simulink model "SlidingModeRobot"  (R2015b)
settings: Solver=ode4  StartTime=0.0  StopTime=20  FixedStep=0.01  RelTol=1e-3
InitFcn:
  | Set_Parameter
StopFcn:
  | Draw_7DOF_FB7roll_point_script
  | DrawResult
values from neighbouring files (symbols this model uses):
  b = 0.1    [Set_Parameter.m]    (also in Set_Parameter_Single.m; Set_Parameter_line_circle.m; Set_Parameter_line_circle_DC_model_no_vision_controller.m; Set_Parameter_sewing_DC_model_no_vision_controller.m)
  J = 0.01    [Set_Parameter.m]    (also in Set_Parameter_Single.m = [0.016,0.016,0.012,0.012,0.01,0.01,0.01]; Set_Parameter_line_circle.m = [0.016,0.016,0.012,0.012,0.01,0.01,0.01]; Set_Parameter_line_circle_DC_model_no_vision_controller.m = [0.016,0.016,0.012,0.012,0.01,0.01,0.01]; Set_Parameter_line_circle_no_vision_controller.m = [10,10,8,8,4,4,4])
  K = 0.01    [Set_Parameter.m]    (also in Set_Parameter_Single.m; Set_Parameter_line_circle.m; Set_Parameter_line_circle_DC_model_no_vision_controller.m; Set_Parameter_sewing_DC_model_no_vision_controller.m)
  L = 0.5    [Set_Parameter.m]    (also in Set_Parameter_Single.m; Set_Parameter_line_circle.m; Set_Parameter_line_circle_DC_model_no_vision_controller.m; Set_Parameter_sewing_DC_model_no_vision_controller.m)
  R = R_z1x2y3(PoseAngle(1),PoseAngle(2),PoseAngle(3))    [IK_7DOF_FB7roll.m]    (also in Set_Parameter.m = 1; Set_Parameter_Single.m = 1; Set_Parameter_line_circle.m = 1; Set_Parameter_line_circle_DC_model_no_vision_controller.m = 1)
undefined symbols (not defined in the file or in its folder): IniJointAngle
libraries: simulink x14
settings Model: Creator=User  LastModifiedBy=User

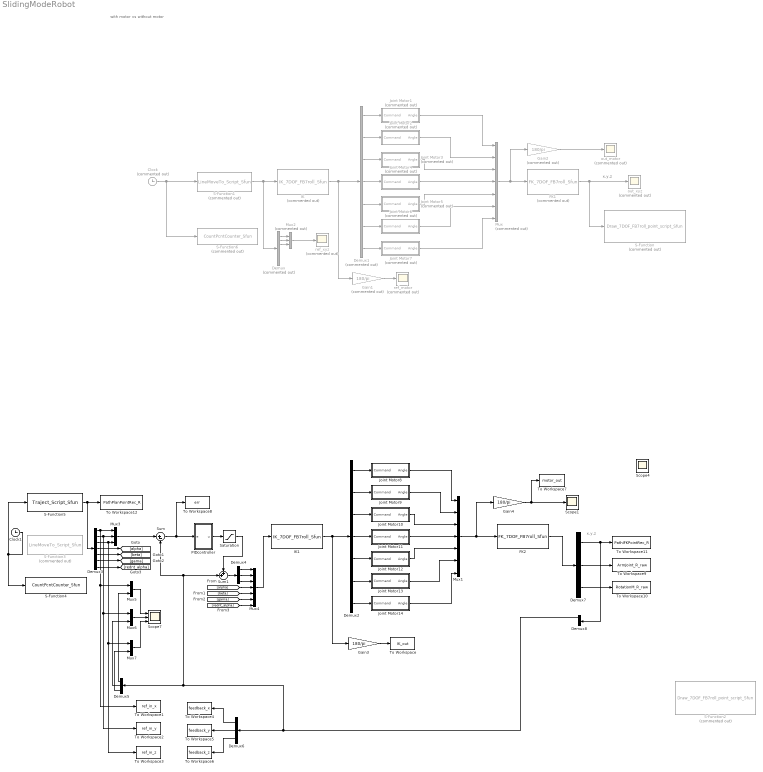
== system SlidingModeRobot ==
  note: with motor vs without motor
  note: x,y,z
  note: x,y,z
  Clock : Clock  Commented=on
  Clock1 : Clock
  Demux : Demux  Commented=on  Outputs=7
  Demux1 : Demux  Commented=on  Outputs=7
  Demux2 : Demux  Outputs=7
  Demux3 : Demux  Outputs=7
  Demux4 : Demux  Outputs=3
  Demux5 : Demux  Outputs=3
  Demux6 : Demux  Outputs=3
  Demux7 : Demux  Outputs=[7,30,9]
  Demux8 : Demux  Outputs=[3,4]
  FK1 : S-Function  Commented=on  FunctionName=FK_7DOF_FB7roll_Sfun  SFunctionDeploymentMode=off  EnableBusSupport=off
  FK2 : S-Function  FunctionName=FK_7DOF_FB7roll_Sfun  SFunctionDeploymentMode=off  EnableBusSupport=off
  Gain1 : Gain  Commented=on  Gain=180/pi
  Gain2 : Gain  Commented=on  Gain=180/pi
  Gain3 : Gain  Gain=180/pi
  Gain4 : Gain  Gain=180/pi
  IK : S-Function  Commented=on  FunctionName=IK_7DOF_FB7roll_Sfun  SFunctionDeploymentMode=off  EnableBusSupport=off
  IK1 : S-Function  FunctionName=IK_7DOF_FB7roll_Sfun  SFunctionDeploymentMode=off  EnableBusSupport=off
  Joint Motor1 : Subsystem  Commented=on
  Joint Motor10 : Subsystem
  Joint Motor11 : Subsystem
  Joint Motor12 : Subsystem
  Joint Motor13 : Subsystem
  Joint Motor14 : Subsystem
  Joint Motor2 : Subsystem  Commented=on
  Joint Motor3 : Subsystem  Commented=on
  Joint Motor4 : Subsystem  Commented=on
  Joint Motor5 : Subsystem  Commented=on
  Joint Motor6 : Subsystem  Commented=on
  Joint Motor7 : Subsystem  Commented=on
  Joint Motor8 : Subsystem
  Joint Motor9 : Subsystem
  Mux : Mux  Commented=on  Inputs=7
  Mux1 : Mux  Inputs=7
  Mux2 : Mux  Commented=on  Inputs=3
  Mux3 : Mux  Inputs=3
  Mux4 : Mux  Inputs=7
  Mux5 : Mux  Inputs=2
  Mux6 : Mux  Inputs=2
  Mux7 : Mux  Inputs=2
  PIDcontroller : Subsystem
  S-Function : S-Function  Commented=on  FunctionName=Draw_7DOF_FB7roll_point_script_Sfun  SFunctionDeploymentMode=off  EnableBusSupport=off
  S-Function1 : S-Function  Commented=on  FunctionName=LineMoveTo_Script_Sfun  SFunctionDeploymentMode=off  EnableBusSupport=off
  S-Function2 : S-Function  Commented=on  FunctionName=Draw_7DOF_FB7roll_point_script_Sfun  SFunctionDeploymentMode=off  EnableBusSupport=off
  S-Function3 : S-Function  Commented=on  FunctionName=LineMoveTo_Script_Sfun  SFunctionDeploymentMode=off  EnableBusSupport=off
  S-Function4 : S-Function  FunctionName=CountPcntCounter_Sfun  SFunctionDeploymentMode=off  EnableBusSupport=off
  S-Function5 : S-Function  FunctionName=Traject_Script_Sfun  SFunctionDeploymentMode=off  EnableBusSupport=off
  S-Function6 : S-Function  Commented=on  FunctionName=CountPcntCounter_Sfun  SFunctionDeploymentMode=off  EnableBusSupport=off
  Saturation : Saturate  UpperLimit=50  LowerLimit=-50
  Scope1 : Scope
  Scope4 : Scope
  Scope7 : Scope  NumInputPorts=3
  Sum : Sum  Inputs=|+-
  Sum1 : Sum  Inputs=++|
  To Workspace : ToWorkspace  VariableName=IK_out  SaveFormat=Timeseries  SampleTime=-1
  To Workspace1 : ToWorkspace  VariableName=ref_in_x  SaveFormat=Timeseries  SampleTime=-1
  To Workspace10 : ToWorkspace  VariableName=RotationM_R_raw  SaveFormat=Timeseries  SampleTime=-1
  To Workspace11 : ToWorkspace  VariableName=PathIFKPointRec_R  SaveFormat=Timeseries  SampleTime=-1
  To Workspace12 : ToWorkspace  VariableName=PathPlanPointRec_R  SaveFormat=Timeseries  SampleTime=-1
  To Workspace2 : ToWorkspace  VariableName=ref_in_y  SaveFormat=Timeseries  SampleTime=-1
  To Workspace3 : ToWorkspace  VariableName=ref_in_z  SaveFormat=Timeseries  SampleTime=-1
  To Workspace4 : ToWorkspace  VariableName=feedback_x  SaveFormat=Timeseries  SampleTime=-1
  To Workspace5 : ToWorkspace  VariableName=feedback_y  SaveFormat=Timeseries  SampleTime=-1
  To Workspace6 : ToWorkspace  VariableName=feedback_z  SaveFormat=Timeseries  SampleTime=-1
  To Workspace7 : ToWorkspace  VariableName=motor_out  SaveFormat=Timeseries  SampleTime=-1
  To Workspace8 : ToWorkspace  VariableName=err  SaveFormat=Timeseries  SampleTime=-1
  To Workspace9 : ToWorkspace  VariableName=ArmJoint_R_raw  SaveFormat=Timeseries  SampleTime=-1
  out_motor : Scope  Commented=on
  out_xyz : Scope  Commented=on
  ref_motor : Scope  Commented=on
  ref_xyz : Scope  Commented=on
  wires:
  Joint Motor3/1(Angle) -> Mux/3
  Joint Motor1/1(Angle) -> Mux/1
  Joint Motor2/1(Angle) -> Mux/2
  Joint Motor4/1(Angle) -> Mux/4
  Joint Motor5/1(Angle) -> Mux/5
  Joint Motor6/1(Angle) -> Mux/6
  Joint Motor7/1(Angle) -> Mux/7
  S-Function1/1 -> Demux/1, IK/1
  Gain1/1 -> ref_motor/1
  FK1/1 -> S-Function/1, out_xyz/1
  Gain2/1 -> out_motor/1
  Demux1/7 -> Joint Motor7/1(Command)
  Demux1/6 -> Joint Motor6/1(Command)
  Demux1/5 -> Joint Motor5/1(Command)
  Demux1/4 -> Joint Motor4/1(Command)
  Demux1/1 -> Joint Motor1/1(Command)
  Demux1/2 -> Joint Motor2/1(Command)
  Demux1/3 -> Joint Motor3/1(Command)
  IK/1 -> Demux1/1, Gain1/1
  Clock/1 -> S-Function6/1, S-Function1/1
  Mux/1 -> Gain2/1, FK1/1
  Joint Motor10/1(Angle) -> Mux1/3
  Joint Motor8/1(Angle) -> Mux1/1
  Joint Motor9/1(Angle) -> Mux1/2
  Joint Motor11/1(Angle) -> Mux1/4
  Joint Motor12/1(Angle) -> Mux1/5
  Joint Motor13/1(Angle) -> Mux1/6
  Joint Motor14/1(Angle) -> Mux1/7
  Gain3/1 -> To Workspace/1
  Gain4/1 -> To Workspace7/1, Scope1/1
  Demux2/7 -> Joint Motor14/1(Command)
  Demux2/6 -> Joint Motor13/1(Command)
  Demux2/5 -> Joint Motor12/1(Command)
  Demux2/4 -> Joint Motor11/1(Command)
  Demux2/1 -> Joint Motor8/1(Command)
  Demux2/2 -> Joint Motor9/1(Command)
  Demux2/3 -> Joint Motor10/1(Command)
  IK1/1 -> Demux2/1, Gain3/1
  Clock1/1 -> S-Function5/1, S-Function4/1
  Mux1/1 -> Gain4/1, FK2/1
  Sum/1 -> To Workspace8/1, PIDcontroller/1(e)
  Demux/1 -> Mux2/1
  Demux/2 -> Mux2/2
  Demux/3 -> Mux2/3
  Mux2/1 -> ref_xyz/1
  Demux3/1 -> Mux3/1, To Workspace1/1, Mux5/1
  Demux3/2 -> Mux3/2, To Workspace2/1, Mux6/1
  Demux3/3 -> Mux7/1, To Workspace3/1, Mux3/3
  Demux3/4 -> [alpha]
  Demux3/5 -> [beta]
  Demux3/6 -> [gama]
  [gama] -> Mux4/6
  [beta] -> Mux4/5
  [alpha] -> Mux4/4
  Demux4/1 -> Mux4/1
  Demux4/2 -> Mux4/2
  Demux4/3 -> Mux4/3
  Mux4/1 -> IK1/1
  Demux3/7 -> [rednt_alpha]
  [rednt_alpha] -> Mux4/7
  S-Function5/1 -> To Workspace12/1, Demux3/1
  Mux3/1 -> Sum/1
  Demux5/1 -> Mux5/2
  Demux5/2 -> Mux6/2
  Demux5/3 -> Mux7/2
  Mux6/1 -> Scope7/2
  Mux5/1 -> Scope7/1
  Mux7/1 -> Scope7/3
  PIDcontroller/1(u) -> Saturation/1
  Saturation/1 -> Sum1/1
  Sum1/1 -> Demux4/1
  Demux6/1 -> To Workspace4/1
  Demux6/2 -> To Workspace5/1
  Demux6/3 -> To Workspace6/1
  FK2/1 -> Demux7/1
  Demux7/1 -> To Workspace11/1, Demux8/1
  Demux7/2 -> To Workspace9/1
  Demux7/3 -> To Workspace10/1
  Demux8/1 -> Sum1/2, Sum/2, Demux5/1, Demux6/1

== system SlidingModeRobot/Joint Motor1 ==
  Command : Inport
  Constant : Constant  Value=IniJointAngle(1)
  DC motor : Subsystem
  Gain : Gain  Gain=30
  Integrator : Integrator  InitialConditionSource=external
  PID Controller : simulink/Continuous/PID Controller  Controller=PID  TimeDomain=Continuous-time  SampleTime=-1  IntegratorMethod=Forward Euler  FilterMethod=Forward Euler  Form=Parallel  UseFilter=on  ControllerParametersSource=internal  P=20  I=0  D=20  N=0  InitialConditionSource=internal  InitialConditionForIntegrator=0  InitialConditionForFilter=0  ExternalReset=none  LimitOutput=off  UpperSaturationLimit=inf  LowerSaturationLimit=-inf  LinearizeAsGain=on  AntiWindupMode=none  Kb=1  TrackingMode=off  Kt=1  PParamMin=[]  PParamMax=[]  IParamMin=[]  IParamMax=[]  DParamMin=[]  DParamMax=[]  NParamMin=[]  NParamMax=[]  KbParamMin=[]  KbParamMax=[]  KtParamMin=[]  KtParamMax=[]  POutMin=[]  POutMax=[]  IOutMin=[]  IOutMax=[]  DOutMin=[]  DOutMax=[]  NOutMin=[]  NOutMax=[]  KbOutMin=[]  KbOutMax=[]  KtOutMin=[]  KtOutMax=[]  IntegratorOutMin=[]  IntegratorOutMax=[]  FilterOutMin=[]  FilterOutMax=[]  SumOutMin=[]  SumOutMax=[]  SumI1OutMin=[]  SumI1OutMax=[]  SumI2OutMin=[]  SumI2OutMax=[]  SumI3OutMin=[]  SumI3OutMax=[]  SumDOutMin=[]  SumDOutMax=[]  SaturationOutMin=[]  SaturationOutMax=[]  IntegratorContinuousStateAttributes=''  IntegratorStateMustResolveToSignalObject=off  IntegratorRTWStateStorageClass=Auto  FilterContinuousStateAttributes=''  FilterStateMustResolveToSignalObject=off  FilterRTWStateStorageClass=Auto  DifferentiatorICPrevScaledInput=0  DifferentiatorOutMin=[]  DifferentiatorOutMax=[]
  Sum : Sum  Inputs=|+-
  Sum1 : Sum  Inputs=|+-
  Angle : Outport
  wires:
  Sum/1 -> PID Controller/1
  PID Controller/1 -> DC motor/1(Voltage)
  DC motor/1(Speed) -> Sum/2, Integrator/1
  Integrator/1 -> Angle/1, Sum1/2
  Command/1 -> Sum1/1
  Sum1/1 -> Gain/1
  Gain/1 -> Sum/1
  Constant/1 -> Integrator/2

== system SlidingModeRobot/Joint Motor10 ==
  Command : Inport
  Constant : Constant  Value=IniJointAngle(3)
  DC motor : Subsystem
  Gain : Gain  Gain=2
  Integrator : Integrator  InitialConditionSource=external
  PID Controller : simulink/Continuous/PID Controller  Controller=PID  TimeDomain=Continuous-time  SampleTime=-1  IntegratorMethod=Forward Euler  FilterMethod=Forward Euler  Form=Parallel  UseFilter=on  ControllerParametersSource=internal  P=20  I=0  D=20  N=0  InitialConditionSource=internal  InitialConditionForIntegrator=0  InitialConditionForFilter=0  ExternalReset=none  LimitOutput=off  UpperSaturationLimit=inf  LowerSaturationLimit=-inf  LinearizeAsGain=on  AntiWindupMode=none  Kb=1  TrackingMode=off  Kt=1  PParamMin=[]  PParamMax=[]  IParamMin=[]  IParamMax=[]  DParamMin=[]  DParamMax=[]  NParamMin=[]  NParamMax=[]  KbParamMin=[]  KbParamMax=[]  KtParamMin=[]  KtParamMax=[]  POutMin=[]  POutMax=[]  IOutMin=[]  IOutMax=[]  DOutMin=[]  DOutMax=[]  NOutMin=[]  NOutMax=[]  KbOutMin=[]  KbOutMax=[]  KtOutMin=[]  KtOutMax=[]  IntegratorOutMin=[]  IntegratorOutMax=[]  FilterOutMin=[]  FilterOutMax=[]  SumOutMin=[]  SumOutMax=[]  SumI1OutMin=[]  SumI1OutMax=[]  SumI2OutMin=[]  SumI2OutMax=[]  SumI3OutMin=[]  SumI3OutMax=[]  SumDOutMin=[]  SumDOutMax=[]  SaturationOutMin=[]  SaturationOutMax=[]  IntegratorContinuousStateAttributes=''  IntegratorStateMustResolveToSignalObject=off  IntegratorRTWStateStorageClass=Auto  FilterContinuousStateAttributes=''  FilterStateMustResolveToSignalObject=off  FilterRTWStateStorageClass=Auto  DifferentiatorICPrevScaledInput=0  DifferentiatorOutMin=[]  DifferentiatorOutMax=[]
  Sum : Sum  Inputs=|+-
  Sum1 : Sum  Inputs=|+-
  Angle : Outport
  wires:
  Sum/1 -> PID Controller/1
  PID Controller/1 -> DC motor/1(Voltage)
  DC motor/1(Speed) -> Sum/2, Integrator/1
  Integrator/1 -> Angle/1, Sum1/2
  Command/1 -> Sum1/1
  Sum1/1 -> Gain/1
  Gain/1 -> Sum/1
  Constant/1 -> Integrator/2

== system SlidingModeRobot/Joint Motor11 ==
  Command : Inport
  Constant : Constant  Value=IniJointAngle(4)
  DC motor : Subsystem
  Gain : Gain  Gain=2
  Integrator : Integrator  InitialConditionSource=external
  PID Controller : simulink/Continuous/PID Controller  Controller=PID  TimeDomain=Continuous-time  SampleTime=-1  IntegratorMethod=Forward Euler  FilterMethod=Forward Euler  Form=Parallel  UseFilter=on  ControllerParametersSource=internal  P=20  I=0  D=20  N=0  InitialConditionSource=internal  InitialConditionForIntegrator=0  InitialConditionForFilter=0  ExternalReset=none  LimitOutput=off  UpperSaturationLimit=inf  LowerSaturationLimit=-inf  LinearizeAsGain=on  AntiWindupMode=none  Kb=1  TrackingMode=off  Kt=1  PParamMin=[]  PParamMax=[]  IParamMin=[]  IParamMax=[]  DParamMin=[]  DParamMax=[]  NParamMin=[]  NParamMax=[]  KbParamMin=[]  KbParamMax=[]  KtParamMin=[]  KtParamMax=[]  POutMin=[]  POutMax=[]  IOutMin=[]  IOutMax=[]  DOutMin=[]  DOutMax=[]  NOutMin=[]  NOutMax=[]  KbOutMin=[]  KbOutMax=[]  KtOutMin=[]  KtOutMax=[]  IntegratorOutMin=[]  IntegratorOutMax=[]  FilterOutMin=[]  FilterOutMax=[]  SumOutMin=[]  SumOutMax=[]  SumI1OutMin=[]  SumI1OutMax=[]  SumI2OutMin=[]  SumI2OutMax=[]  SumI3OutMin=[]  SumI3OutMax=[]  SumDOutMin=[]  SumDOutMax=[]  SaturationOutMin=[]  SaturationOutMax=[]  IntegratorContinuousStateAttributes=''  IntegratorStateMustResolveToSignalObject=off  IntegratorRTWStateStorageClass=Auto  FilterContinuousStateAttributes=''  FilterStateMustResolveToSignalObject=off  FilterRTWStateStorageClass=Auto  DifferentiatorICPrevScaledInput=0  DifferentiatorOutMin=[]  DifferentiatorOutMax=[]
  Sum : Sum  Inputs=|+-
  Sum1 : Sum  Inputs=|+-
  Angle : Outport
  wires:
  Sum/1 -> PID Controller/1
  PID Controller/1 -> DC motor/1(Voltage)
  DC motor/1(Speed) -> Sum/2, Integrator/1
  Integrator/1 -> Angle/1, Sum1/2
  Command/1 -> Sum1/1
  Sum1/1 -> Gain/1
  Gain/1 -> Sum/1
  Constant/1 -> Integrator/2

== system SlidingModeRobot/Joint Motor12 ==
  Command : Inport
  Constant : Constant  Value=IniJointAngle(5)
  DC motor : Subsystem
  Gain : Gain  Gain=2
  Integrator : Integrator  InitialConditionSource=external
  PID Controller : simulink/Continuous/PID Controller  Controller=PID  TimeDomain=Continuous-time  SampleTime=-1  IntegratorMethod=Forward Euler  FilterMethod=Forward Euler  Form=Parallel  UseFilter=on  ControllerParametersSource=internal  P=20  I=0  D=20  N=0  InitialConditionSource=internal  InitialConditionForIntegrator=0  InitialConditionForFilter=0  ExternalReset=none  LimitOutput=off  UpperSaturationLimit=inf  LowerSaturationLimit=-inf  LinearizeAsGain=on  AntiWindupMode=none  Kb=1  TrackingMode=off  Kt=1  PParamMin=[]  PParamMax=[]  IParamMin=[]  IParamMax=[]  DParamMin=[]  DParamMax=[]  NParamMin=[]  NParamMax=[]  KbParamMin=[]  KbParamMax=[]  KtParamMin=[]  KtParamMax=[]  POutMin=[]  POutMax=[]  IOutMin=[]  IOutMax=[]  DOutMin=[]  DOutMax=[]  NOutMin=[]  NOutMax=[]  KbOutMin=[]  KbOutMax=[]  KtOutMin=[]  KtOutMax=[]  IntegratorOutMin=[]  IntegratorOutMax=[]  FilterOutMin=[]  FilterOutMax=[]  SumOutMin=[]  SumOutMax=[]  SumI1OutMin=[]  SumI1OutMax=[]  SumI2OutMin=[]  SumI2OutMax=[]  SumI3OutMin=[]  SumI3OutMax=[]  SumDOutMin=[]  SumDOutMax=[]  SaturationOutMin=[]  SaturationOutMax=[]  IntegratorContinuousStateAttributes=''  IntegratorStateMustResolveToSignalObject=off  IntegratorRTWStateStorageClass=Auto  FilterContinuousStateAttributes=''  FilterStateMustResolveToSignalObject=off  FilterRTWStateStorageClass=Auto  DifferentiatorICPrevScaledInput=0  DifferentiatorOutMin=[]  DifferentiatorOutMax=[]
  Sum : Sum  Inputs=|+-
  Sum1 : Sum  Inputs=|+-
  Angle : Outport
  wires:
  Sum/1 -> PID Controller/1
  PID Controller/1 -> DC motor/1(Voltage)
  DC motor/1(Speed) -> Sum/2, Integrator/1
  Integrator/1 -> Angle/1, Sum1/2
  Command/1 -> Sum1/1
  Sum1/1 -> Gain/1
  Gain/1 -> Sum/1
  Constant/1 -> Integrator/2

== system SlidingModeRobot/Joint Motor13 ==
  Command : Inport
  Constant : Constant  Value=IniJointAngle(6)
  DC motor : Subsystem
  Gain : Gain  Gain=2
  Integrator : Integrator  InitialConditionSource=external
  PID Controller : simulink/Continuous/PID Controller  Controller=PID  TimeDomain=Continuous-time  SampleTime=-1  IntegratorMethod=Forward Euler  FilterMethod=Forward Euler  Form=Parallel  UseFilter=on  ControllerParametersSource=internal  P=20  I=0  D=20  N=0  InitialConditionSource=internal  InitialConditionForIntegrator=0  InitialConditionForFilter=0  ExternalReset=none  LimitOutput=off  UpperSaturationLimit=inf  LowerSaturationLimit=-inf  LinearizeAsGain=on  AntiWindupMode=none  Kb=1  TrackingMode=off  Kt=1  PParamMin=[]  PParamMax=[]  IParamMin=[]  IParamMax=[]  DParamMin=[]  DParamMax=[]  NParamMin=[]  NParamMax=[]  KbParamMin=[]  KbParamMax=[]  KtParamMin=[]  KtParamMax=[]  POutMin=[]  POutMax=[]  IOutMin=[]  IOutMax=[]  DOutMin=[]  DOutMax=[]  NOutMin=[]  NOutMax=[]  KbOutMin=[]  KbOutMax=[]  KtOutMin=[]  KtOutMax=[]  IntegratorOutMin=[]  IntegratorOutMax=[]  FilterOutMin=[]  FilterOutMax=[]  SumOutMin=[]  SumOutMax=[]  SumI1OutMin=[]  SumI1OutMax=[]  SumI2OutMin=[]  SumI2OutMax=[]  SumI3OutMin=[]  SumI3OutMax=[]  SumDOutMin=[]  SumDOutMax=[]  SaturationOutMin=[]  SaturationOutMax=[]  IntegratorContinuousStateAttributes=''  IntegratorStateMustResolveToSignalObject=off  IntegratorRTWStateStorageClass=Auto  FilterContinuousStateAttributes=''  FilterStateMustResolveToSignalObject=off  FilterRTWStateStorageClass=Auto  DifferentiatorICPrevScaledInput=0  DifferentiatorOutMin=[]  DifferentiatorOutMax=[]
  Sum : Sum  Inputs=|+-
  Sum1 : Sum  Inputs=|+-
  Angle : Outport
  wires:
  Sum/1 -> PID Controller/1
  PID Controller/1 -> DC motor/1(Voltage)
  DC motor/1(Speed) -> Sum/2, Integrator/1
  Integrator/1 -> Angle/1, Sum1/2
  Command/1 -> Sum1/1
  Sum1/1 -> Gain/1
  Gain/1 -> Sum/1
  Constant/1 -> Integrator/2

== system SlidingModeRobot/Joint Motor14 ==
  Command : Inport
  Constant : Constant  Value=IniJointAngle(7)
  DC motor : Subsystem
  Gain : Gain  Gain=2
  Integrator : Integrator  InitialConditionSource=external
  PID Controller : simulink/Continuous/PID Controller  Controller=PID  TimeDomain=Continuous-time  SampleTime=-1  IntegratorMethod=Forward Euler  FilterMethod=Forward Euler  Form=Parallel  UseFilter=on  ControllerParametersSource=internal  P=20  I=0  D=20  N=0  InitialConditionSource=internal  InitialConditionForIntegrator=0  InitialConditionForFilter=0  ExternalReset=none  LimitOutput=off  UpperSaturationLimit=inf  LowerSaturationLimit=-inf  LinearizeAsGain=on  AntiWindupMode=none  Kb=1  TrackingMode=off  Kt=1  PParamMin=[]  PParamMax=[]  IParamMin=[]  IParamMax=[]  DParamMin=[]  DParamMax=[]  NParamMin=[]  NParamMax=[]  KbParamMin=[]  KbParamMax=[]  KtParamMin=[]  KtParamMax=[]  POutMin=[]  POutMax=[]  IOutMin=[]  IOutMax=[]  DOutMin=[]  DOutMax=[]  NOutMin=[]  NOutMax=[]  KbOutMin=[]  KbOutMax=[]  KtOutMin=[]  KtOutMax=[]  IntegratorOutMin=[]  IntegratorOutMax=[]  FilterOutMin=[]  FilterOutMax=[]  SumOutMin=[]  SumOutMax=[]  SumI1OutMin=[]  SumI1OutMax=[]  SumI2OutMin=[]  SumI2OutMax=[]  SumI3OutMin=[]  SumI3OutMax=[]  SumDOutMin=[]  SumDOutMax=[]  SaturationOutMin=[]  SaturationOutMax=[]  IntegratorContinuousStateAttributes=''  IntegratorStateMustResolveToSignalObject=off  IntegratorRTWStateStorageClass=Auto  FilterContinuousStateAttributes=''  FilterStateMustResolveToSignalObject=off  FilterRTWStateStorageClass=Auto  DifferentiatorICPrevScaledInput=0  DifferentiatorOutMin=[]  DifferentiatorOutMax=[]
  Sum : Sum  Inputs=|+-
  Sum1 : Sum  Inputs=|+-
  Angle : Outport
  wires:
  Sum/1 -> PID Controller/1
  PID Controller/1 -> DC motor/1(Voltage)
  DC motor/1(Speed) -> Sum/2, Integrator/1
  Integrator/1 -> Angle/1, Sum1/2
  Command/1 -> Sum1/1
  Sum1/1 -> Gain/1
  Gain/1 -> Sum/1
  Constant/1 -> Integrator/2

== system SlidingModeRobot/Joint Motor2 ==
  Command : Inport
  Constant : Constant  Value=IniJointAngle(2)
  DC motor : Subsystem
  Gain : Gain  Gain=32
  Integrator : Integrator  InitialConditionSource=external
  PID Controller : simulink/Continuous/PID Controller  Controller=PID  TimeDomain=Continuous-time  SampleTime=-1  IntegratorMethod=Forward Euler  FilterMethod=Forward Euler  Form=Parallel  UseFilter=on  ControllerParametersSource=internal  P=20  I=0  D=20  N=0  InitialConditionSource=internal  InitialConditionForIntegrator=0  InitialConditionForFilter=0  ExternalReset=none  LimitOutput=off  UpperSaturationLimit=inf  LowerSaturationLimit=-inf  LinearizeAsGain=on  AntiWindupMode=none  Kb=1  TrackingMode=off  Kt=1  PParamMin=[]  PParamMax=[]  IParamMin=[]  IParamMax=[]  DParamMin=[]  DParamMax=[]  NParamMin=[]  NParamMax=[]  KbParamMin=[]  KbParamMax=[]  KtParamMin=[]  KtParamMax=[]  POutMin=[]  POutMax=[]  IOutMin=[]  IOutMax=[]  DOutMin=[]  DOutMax=[]  NOutMin=[]  NOutMax=[]  KbOutMin=[]  KbOutMax=[]  KtOutMin=[]  KtOutMax=[]  IntegratorOutMin=[]  IntegratorOutMax=[]  FilterOutMin=[]  FilterOutMax=[]  SumOutMin=[]  SumOutMax=[]  SumI1OutMin=[]  SumI1OutMax=[]  SumI2OutMin=[]  SumI2OutMax=[]  SumI3OutMin=[]  SumI3OutMax=[]  SumDOutMin=[]  SumDOutMax=[]  SaturationOutMin=[]  SaturationOutMax=[]  IntegratorContinuousStateAttributes=''  IntegratorStateMustResolveToSignalObject=off  IntegratorRTWStateStorageClass=Auto  FilterContinuousStateAttributes=''  FilterStateMustResolveToSignalObject=off  FilterRTWStateStorageClass=Auto  DifferentiatorICPrevScaledInput=0  DifferentiatorOutMin=[]  DifferentiatorOutMax=[]
  Sum : Sum  Inputs=|+-
  Sum1 : Sum  Inputs=|+-
  Angle : Outport
  wires:
  Sum/1 -> PID Controller/1
  PID Controller/1 -> DC motor/1(Voltage)
  DC motor/1(Speed) -> Sum/2, Integrator/1
  Integrator/1 -> Angle/1, Sum1/2
  Command/1 -> Sum1/1
  Sum1/1 -> Gain/1
  Gain/1 -> Sum/1
  Constant/1 -> Integrator/2

== system SlidingModeRobot/Joint Motor3 ==
  Command : Inport
  Constant : Constant  Value=IniJointAngle(3)
  DC motor : Subsystem
  Gain : Gain  Gain=30
  Integrator : Integrator  InitialConditionSource=external
  PID Controller : simulink/Continuous/PID Controller  Controller=PID  TimeDomain=Continuous-time  SampleTime=-1  IntegratorMethod=Forward Euler  FilterMethod=Forward Euler  Form=Parallel  UseFilter=on  ControllerParametersSource=internal  P=20  I=0  D=20  N=0  InitialConditionSource=internal  InitialConditionForIntegrator=0  InitialConditionForFilter=0  ExternalReset=none  LimitOutput=off  UpperSaturationLimit=inf  LowerSaturationLimit=-inf  LinearizeAsGain=on  AntiWindupMode=none  Kb=1  TrackingMode=off  Kt=1  PParamMin=[]  PParamMax=[]  IParamMin=[]  IParamMax=[]  DParamMin=[]  DParamMax=[]  NParamMin=[]  NParamMax=[]  KbParamMin=[]  KbParamMax=[]  KtParamMin=[]  KtParamMax=[]  POutMin=[]  POutMax=[]  IOutMin=[]  IOutMax=[]  DOutMin=[]  DOutMax=[]  NOutMin=[]  NOutMax=[]  KbOutMin=[]  KbOutMax=[]  KtOutMin=[]  KtOutMax=[]  IntegratorOutMin=[]  IntegratorOutMax=[]  FilterOutMin=[]  FilterOutMax=[]  SumOutMin=[]  SumOutMax=[]  SumI1OutMin=[]  SumI1OutMax=[]  SumI2OutMin=[]  SumI2OutMax=[]  SumI3OutMin=[]  SumI3OutMax=[]  SumDOutMin=[]  SumDOutMax=[]  SaturationOutMin=[]  SaturationOutMax=[]  IntegratorContinuousStateAttributes=''  IntegratorStateMustResolveToSignalObject=off  IntegratorRTWStateStorageClass=Auto  FilterContinuousStateAttributes=''  FilterStateMustResolveToSignalObject=off  FilterRTWStateStorageClass=Auto  DifferentiatorICPrevScaledInput=0  DifferentiatorOutMin=[]  DifferentiatorOutMax=[]
  Sum : Sum  Inputs=|+-
  Sum1 : Sum  Inputs=|+-
  Angle : Outport
  wires:
  Sum/1 -> PID Controller/1
  PID Controller/1 -> DC motor/1(Voltage)
  DC motor/1(Speed) -> Sum/2, Integrator/1
  Integrator/1 -> Angle/1, Sum1/2
  Command/1 -> Sum1/1
  Sum1/1 -> Gain/1
  Gain/1 -> Sum/1
  Constant/1 -> Integrator/2

== system SlidingModeRobot/Joint Motor4 ==
  Command : Inport
  Constant : Constant  Value=IniJointAngle(4)
  DC motor : Subsystem
  Gain : Gain  Gain=10
  Integrator : Integrator  InitialConditionSource=external
  PID Controller : simulink/Continuous/PID Controller  Controller=PID  TimeDomain=Continuous-time  SampleTime=-1  IntegratorMethod=Forward Euler  FilterMethod=Forward Euler  Form=Parallel  UseFilter=on  ControllerParametersSource=internal  P=20  I=0  D=20  N=0  InitialConditionSource=internal  InitialConditionForIntegrator=0  InitialConditionForFilter=0  ExternalReset=none  LimitOutput=off  UpperSaturationLimit=inf  LowerSaturationLimit=-inf  LinearizeAsGain=on  AntiWindupMode=none  Kb=1  TrackingMode=off  Kt=1  PParamMin=[]  PParamMax=[]  IParamMin=[]  IParamMax=[]  DParamMin=[]  DParamMax=[]  NParamMin=[]  NParamMax=[]  KbParamMin=[]  KbParamMax=[]  KtParamMin=[]  KtParamMax=[]  POutMin=[]  POutMax=[]  IOutMin=[]  IOutMax=[]  DOutMin=[]  DOutMax=[]  NOutMin=[]  NOutMax=[]  KbOutMin=[]  KbOutMax=[]  KtOutMin=[]  KtOutMax=[]  IntegratorOutMin=[]  IntegratorOutMax=[]  FilterOutMin=[]  FilterOutMax=[]  SumOutMin=[]  SumOutMax=[]  SumI1OutMin=[]  SumI1OutMax=[]  SumI2OutMin=[]  SumI2OutMax=[]  SumI3OutMin=[]  SumI3OutMax=[]  SumDOutMin=[]  SumDOutMax=[]  SaturationOutMin=[]  SaturationOutMax=[]  IntegratorContinuousStateAttributes=''  IntegratorStateMustResolveToSignalObject=off  IntegratorRTWStateStorageClass=Auto  FilterContinuousStateAttributes=''  FilterStateMustResolveToSignalObject=off  FilterRTWStateStorageClass=Auto  DifferentiatorICPrevScaledInput=0  DifferentiatorOutMin=[]  DifferentiatorOutMax=[]
  Sum : Sum  Inputs=|+-
  Sum1 : Sum  Inputs=|+-
  Angle : Outport
  wires:
  Sum/1 -> PID Controller/1
  PID Controller/1 -> DC motor/1(Voltage)
  DC motor/1(Speed) -> Sum/2, Integrator/1
  Integrator/1 -> Angle/1, Sum1/2
  Command/1 -> Sum1/1
  Sum1/1 -> Gain/1
  Gain/1 -> Sum/1
  Constant/1 -> Integrator/2

== system SlidingModeRobot/Joint Motor5 ==
  Command : Inport
  Constant : Constant  Value=IniJointAngle(5)
  DC motor : Subsystem
  Gain : Gain  Gain=2
  Integrator : Integrator  InitialConditionSource=external
  PID Controller : simulink/Continuous/PID Controller  Controller=PID  TimeDomain=Continuous-time  SampleTime=-1  IntegratorMethod=Forward Euler  FilterMethod=Forward Euler  Form=Parallel  UseFilter=on  ControllerParametersSource=internal  P=20  I=0  D=20  N=0  InitialConditionSource=internal  InitialConditionForIntegrator=0  InitialConditionForFilter=0  ExternalReset=none  LimitOutput=off  UpperSaturationLimit=inf  LowerSaturationLimit=-inf  LinearizeAsGain=on  AntiWindupMode=none  Kb=1  TrackingMode=off  Kt=1  PParamMin=[]  PParamMax=[]  IParamMin=[]  IParamMax=[]  DParamMin=[]  DParamMax=[]  NParamMin=[]  NParamMax=[]  KbParamMin=[]  KbParamMax=[]  KtParamMin=[]  KtParamMax=[]  POutMin=[]  POutMax=[]  IOutMin=[]  IOutMax=[]  DOutMin=[]  DOutMax=[]  NOutMin=[]  NOutMax=[]  KbOutMin=[]  KbOutMax=[]  KtOutMin=[]  KtOutMax=[]  IntegratorOutMin=[]  IntegratorOutMax=[]  FilterOutMin=[]  FilterOutMax=[]  SumOutMin=[]  SumOutMax=[]  SumI1OutMin=[]  SumI1OutMax=[]  SumI2OutMin=[]  SumI2OutMax=[]  SumI3OutMin=[]  SumI3OutMax=[]  SumDOutMin=[]  SumDOutMax=[]  SaturationOutMin=[]  SaturationOutMax=[]  IntegratorContinuousStateAttributes=''  IntegratorStateMustResolveToSignalObject=off  IntegratorRTWStateStorageClass=Auto  FilterContinuousStateAttributes=''  FilterStateMustResolveToSignalObject=off  FilterRTWStateStorageClass=Auto  DifferentiatorICPrevScaledInput=0  DifferentiatorOutMin=[]  DifferentiatorOutMax=[]
  Sum : Sum  Inputs=|+-
  Sum1 : Sum  Inputs=|+-
  Angle : Outport
  wires:
  Sum/1 -> PID Controller/1
  PID Controller/1 -> DC motor/1(Voltage)
  DC motor/1(Speed) -> Sum/2, Integrator/1
  Integrator/1 -> Angle/1, Sum1/2
  Command/1 -> Sum1/1
  Sum1/1 -> Gain/1
  Gain/1 -> Sum/1
  Constant/1 -> Integrator/2

== system SlidingModeRobot/Joint Motor6 ==
  Command : Inport
  Constant : Constant  Value=IniJointAngle(6)
  DC motor : Subsystem
  Gain : Gain  Gain=2
  Integrator : Integrator  InitialConditionSource=external
  PID Controller : simulink/Continuous/PID Controller  Controller=PID  TimeDomain=Continuous-time  SampleTime=-1  IntegratorMethod=Forward Euler  FilterMethod=Forward Euler  Form=Parallel  UseFilter=on  ControllerParametersSource=internal  P=20  I=0  D=20  N=0  InitialConditionSource=internal  InitialConditionForIntegrator=0  InitialConditionForFilter=0  ExternalReset=none  LimitOutput=off  UpperSaturationLimit=inf  LowerSaturationLimit=-inf  LinearizeAsGain=on  AntiWindupMode=none  Kb=1  TrackingMode=off  Kt=1  PParamMin=[]  PParamMax=[]  IParamMin=[]  IParamMax=[]  DParamMin=[]  DParamMax=[]  NParamMin=[]  NParamMax=[]  KbParamMin=[]  KbParamMax=[]  KtParamMin=[]  KtParamMax=[]  POutMin=[]  POutMax=[]  IOutMin=[]  IOutMax=[]  DOutMin=[]  DOutMax=[]  NOutMin=[]  NOutMax=[]  KbOutMin=[]  KbOutMax=[]  KtOutMin=[]  KtOutMax=[]  IntegratorOutMin=[]  IntegratorOutMax=[]  FilterOutMin=[]  FilterOutMax=[]  SumOutMin=[]  SumOutMax=[]  SumI1OutMin=[]  SumI1OutMax=[]  SumI2OutMin=[]  SumI2OutMax=[]  SumI3OutMin=[]  SumI3OutMax=[]  SumDOutMin=[]  SumDOutMax=[]  SaturationOutMin=[]  SaturationOutMax=[]  IntegratorContinuousStateAttributes=''  IntegratorStateMustResolveToSignalObject=off  IntegratorRTWStateStorageClass=Auto  FilterContinuousStateAttributes=''  FilterStateMustResolveToSignalObject=off  FilterRTWStateStorageClass=Auto  DifferentiatorICPrevScaledInput=0  DifferentiatorOutMin=[]  DifferentiatorOutMax=[]
  Sum : Sum  Inputs=|+-
  Sum1 : Sum  Inputs=|+-
  Angle : Outport
  wires:
  Sum/1 -> PID Controller/1
  PID Controller/1 -> DC motor/1(Voltage)
  DC motor/1(Speed) -> Sum/2, Integrator/1
  Integrator/1 -> Angle/1, Sum1/2
  Command/1 -> Sum1/1
  Sum1/1 -> Gain/1
  Gain/1 -> Sum/1
  Constant/1 -> Integrator/2

== system SlidingModeRobot/Joint Motor7 ==
  Command : Inport
  Constant : Constant  Value=IniJointAngle(7)
  DC motor : Subsystem
  Gain : Gain  Gain=2
  Integrator : Integrator  InitialConditionSource=external
  PID Controller : simulink/Continuous/PID Controller  Controller=PID  TimeDomain=Continuous-time  SampleTime=-1  IntegratorMethod=Forward Euler  FilterMethod=Forward Euler  Form=Parallel  UseFilter=on  ControllerParametersSource=internal  P=20  I=0  D=20  N=0  InitialConditionSource=internal  InitialConditionForIntegrator=0  InitialConditionForFilter=0  ExternalReset=none  LimitOutput=off  UpperSaturationLimit=inf  LowerSaturationLimit=-inf  LinearizeAsGain=on  AntiWindupMode=none  Kb=1  TrackingMode=off  Kt=1  PParamMin=[]  PParamMax=[]  IParamMin=[]  IParamMax=[]  DParamMin=[]  DParamMax=[]  NParamMin=[]  NParamMax=[]  KbParamMin=[]  KbParamMax=[]  KtParamMin=[]  KtParamMax=[]  POutMin=[]  POutMax=[]  IOutMin=[]  IOutMax=[]  DOutMin=[]  DOutMax=[]  NOutMin=[]  NOutMax=[]  KbOutMin=[]  KbOutMax=[]  KtOutMin=[]  KtOutMax=[]  IntegratorOutMin=[]  IntegratorOutMax=[]  FilterOutMin=[]  FilterOutMax=[]  SumOutMin=[]  SumOutMax=[]  SumI1OutMin=[]  SumI1OutMax=[]  SumI2OutMin=[]  SumI2OutMax=[]  SumI3OutMin=[]  SumI3OutMax=[]  SumDOutMin=[]  SumDOutMax=[]  SaturationOutMin=[]  SaturationOutMax=[]  IntegratorContinuousStateAttributes=''  IntegratorStateMustResolveToSignalObject=off  IntegratorRTWStateStorageClass=Auto  FilterContinuousStateAttributes=''  FilterStateMustResolveToSignalObject=off  FilterRTWStateStorageClass=Auto  DifferentiatorICPrevScaledInput=0  DifferentiatorOutMin=[]  DifferentiatorOutMax=[]
  Sum : Sum  Inputs=|+-
  Sum1 : Sum  Inputs=|+-
  Angle : Outport
  wires:
  Sum/1 -> PID Controller/1
  PID Controller/1 -> DC motor/1(Voltage)
  DC motor/1(Speed) -> Sum/2, Integrator/1
  Integrator/1 -> Angle/1, Sum1/2
  Command/1 -> Sum1/1
  Sum1/1 -> Gain/1
  Gain/1 -> Sum/1
  Constant/1 -> Integrator/2

== system SlidingModeRobot/Joint Motor8 ==
  Command : Inport
  Constant : Constant  Value=IniJointAngle(1)
  DC motor : Subsystem
  Gain : Gain  Gain=2
  Integrator : Integrator  InitialConditionSource=external
  PID Controller : simulink/Continuous/PID Controller  Controller=PID  TimeDomain=Continuous-time  SampleTime=-1  IntegratorMethod=Forward Euler  FilterMethod=Forward Euler  Form=Parallel  UseFilter=on  ControllerParametersSource=internal  P=20  I=0  D=20  N=0  InitialConditionSource=internal  InitialConditionForIntegrator=0  InitialConditionForFilter=0  ExternalReset=none  LimitOutput=off  UpperSaturationLimit=inf  LowerSaturationLimit=-inf  LinearizeAsGain=on  AntiWindupMode=none  Kb=1  TrackingMode=off  Kt=1  PParamMin=[]  PParamMax=[]  IParamMin=[]  IParamMax=[]  DParamMin=[]  DParamMax=[]  NParamMin=[]  NParamMax=[]  KbParamMin=[]  KbParamMax=[]  KtParamMin=[]  KtParamMax=[]  POutMin=[]  POutMax=[]  IOutMin=[]  IOutMax=[]  DOutMin=[]  DOutMax=[]  NOutMin=[]  NOutMax=[]  KbOutMin=[]  KbOutMax=[]  KtOutMin=[]  KtOutMax=[]  IntegratorOutMin=[]  IntegratorOutMax=[]  FilterOutMin=[]  FilterOutMax=[]  SumOutMin=[]  SumOutMax=[]  SumI1OutMin=[]  SumI1OutMax=[]  SumI2OutMin=[]  SumI2OutMax=[]  SumI3OutMin=[]  SumI3OutMax=[]  SumDOutMin=[]  SumDOutMax=[]  SaturationOutMin=[]  SaturationOutMax=[]  IntegratorContinuousStateAttributes=''  IntegratorStateMustResolveToSignalObject=off  IntegratorRTWStateStorageClass=Auto  FilterContinuousStateAttributes=''  FilterStateMustResolveToSignalObject=off  FilterRTWStateStorageClass=Auto  DifferentiatorICPrevScaledInput=0  DifferentiatorOutMin=[]  DifferentiatorOutMax=[]
  Sum : Sum  Inputs=|+-
  Sum1 : Sum  Inputs=|+-
  Angle : Outport
  wires:
  Sum/1 -> PID Controller/1
  PID Controller/1 -> DC motor/1(Voltage)
  DC motor/1(Speed) -> Sum/2, Integrator/1
  Integrator/1 -> Angle/1, Sum1/2
  Command/1 -> Sum1/1
  Sum1/1 -> Gain/1
  Gain/1 -> Sum/1
  Constant/1 -> Integrator/2

== system SlidingModeRobot/Joint Motor9 ==
  Command : Inport
  Constant : Constant  Value=IniJointAngle(2)
  DC motor : Subsystem
  Gain : Gain  Gain=2
  Integrator : Integrator  InitialConditionSource=external
  PID Controller : simulink/Continuous/PID Controller  Controller=PID  TimeDomain=Continuous-time  SampleTime=-1  IntegratorMethod=Forward Euler  FilterMethod=Forward Euler  Form=Parallel  UseFilter=on  ControllerParametersSource=internal  P=20  I=0  D=20  N=0  InitialConditionSource=internal  InitialConditionForIntegrator=0  InitialConditionForFilter=0  ExternalReset=none  LimitOutput=off  UpperSaturationLimit=inf  LowerSaturationLimit=-inf  LinearizeAsGain=on  AntiWindupMode=none  Kb=1  TrackingMode=off  Kt=1  PParamMin=[]  PParamMax=[]  IParamMin=[]  IParamMax=[]  DParamMin=[]  DParamMax=[]  NParamMin=[]  NParamMax=[]  KbParamMin=[]  KbParamMax=[]  KtParamMin=[]  KtParamMax=[]  POutMin=[]  POutMax=[]  IOutMin=[]  IOutMax=[]  DOutMin=[]  DOutMax=[]  NOutMin=[]  NOutMax=[]  KbOutMin=[]  KbOutMax=[]  KtOutMin=[]  KtOutMax=[]  IntegratorOutMin=[]  IntegratorOutMax=[]  FilterOutMin=[]  FilterOutMax=[]  SumOutMin=[]  SumOutMax=[]  SumI1OutMin=[]  SumI1OutMax=[]  SumI2OutMin=[]  SumI2OutMax=[]  SumI3OutMin=[]  SumI3OutMax=[]  SumDOutMin=[]  SumDOutMax=[]  SaturationOutMin=[]  SaturationOutMax=[]  IntegratorContinuousStateAttributes=''  IntegratorStateMustResolveToSignalObject=off  IntegratorRTWStateStorageClass=Auto  FilterContinuousStateAttributes=''  FilterStateMustResolveToSignalObject=off  FilterRTWStateStorageClass=Auto  DifferentiatorICPrevScaledInput=0  DifferentiatorOutMin=[]  DifferentiatorOutMax=[]
  Sum : Sum  Inputs=|+-
  Sum1 : Sum  Inputs=|+-
  Angle : Outport
  wires:
  Sum/1 -> PID Controller/1
  PID Controller/1 -> DC motor/1(Voltage)
  DC motor/1(Speed) -> Sum/2, Integrator/1
  Integrator/1 -> Angle/1, Sum1/2
  Command/1 -> Sum1/1
  Sum1/1 -> Gain/1
  Gain/1 -> Sum/1
  Constant/1 -> Integrator/2

== system SlidingModeRobot/PIDcontroller ==
  e : Inport
  D gain : Gain  Gain=0.9
  D scope : Scope
  Derivative : Derivative
  I gain : Gain  Gain=1.3
  I scope : Scope
  Integrator : Integrator
  P gain : Gain  Gain=8
  P scope : Scope
  Sum1 : Sum  Inputs=+++
  u : Outport
  wires:
  I gain/1 -> Integrator/1
  P gain/1 -> P scope/1, Sum1/1
  Integrator/1 -> I scope/1, Sum1/2
  e/1 -> D gain/1, I gain/1, P gain/1
  Sum1/1 -> u/1
  D gain/1 -> Derivative/1
  Derivative/1 -> D scope/1, Sum1/3

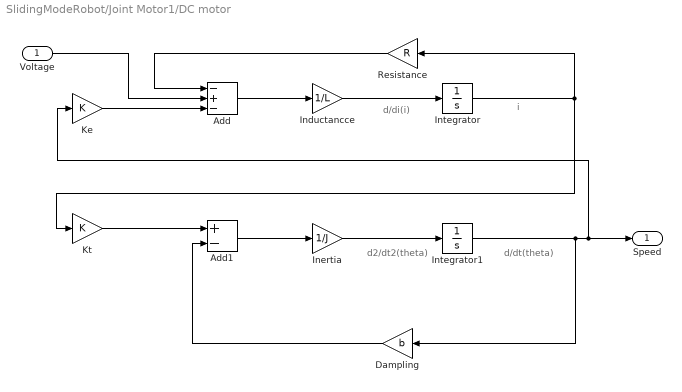
== system SlidingModeRobot/Joint Motor1/DC motor ==
  note: d/dt(theta)
  note: d2/dt2(theta)
  note: i
  note: d/di(i)
  Voltage : Inport
  Add : Sum  Inputs=-+-
  Add1 : Sum  Inputs=+-
  Dampling : Gain  Gain=b
  Inductancce : Gain  Gain=1/L
  Inertia : Gain  Gain=1/J
  Integrator : Integrator
  Integrator1 : Integrator
  Ke : Gain  Gain=K
  Kt : Gain  Gain=K
  Resistance : Gain  Gain=R
  Speed : Outport
  wires:
  Resistance/1 -> Add/1
  Add/1 -> Inductancce/1
  Inductancce/1 -> Integrator/1
  Inertia/1 -> Integrator1/1
  Kt/1 -> Add1/1
  Add1/1 -> Inertia/1
  Integrator/1 -> Kt/1, Resistance/1
  Voltage/1 -> Add/2
  Dampling/1 -> Add1/2
  Integrator1/1 -> Dampling/1, Speed/1, Ke/1
  Ke/1 -> Add/3

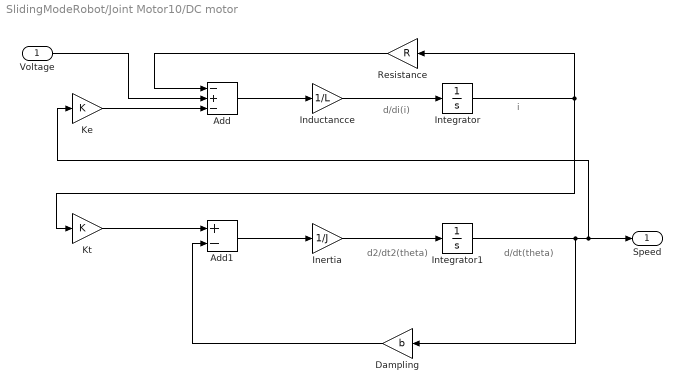
== system SlidingModeRobot/Joint Motor10/DC motor ==
  note: d/dt(theta)
  note: d2/dt2(theta)
  note: i
  note: d/di(i)
  Voltage : Inport
  Add : Sum  Inputs=-+-
  Add1 : Sum  Inputs=+-
  Dampling : Gain  Gain=b
  Inductancce : Gain  Gain=1/L
  Inertia : Gain  Gain=1/J
  Integrator : Integrator
  Integrator1 : Integrator
  Ke : Gain  Gain=K
  Kt : Gain  Gain=K
  Resistance : Gain  Gain=R
  Speed : Outport
  wires:
  Resistance/1 -> Add/1
  Add/1 -> Inductancce/1
  Inductancce/1 -> Integrator/1
  Inertia/1 -> Integrator1/1
  Kt/1 -> Add1/1
  Add1/1 -> Inertia/1
  Integrator/1 -> Kt/1, Resistance/1
  Voltage/1 -> Add/2
  Dampling/1 -> Add1/2
  Integrator1/1 -> Dampling/1, Speed/1, Ke/1
  Ke/1 -> Add/3

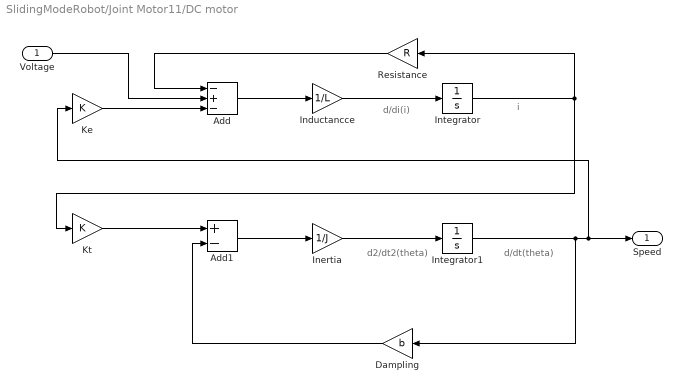
== system SlidingModeRobot/Joint Motor11/DC motor ==
  note: d/dt(theta)
  note: d2/dt2(theta)
  note: i
  note: d/di(i)
  Voltage : Inport
  Add : Sum  Inputs=-+-
  Add1 : Sum  Inputs=+-
  Dampling : Gain  Gain=b
  Inductancce : Gain  Gain=1/L
  Inertia : Gain  Gain=1/J
  Integrator : Integrator
  Integrator1 : Integrator
  Ke : Gain  Gain=K
  Kt : Gain  Gain=K
  Resistance : Gain  Gain=R
  Speed : Outport
  wires:
  Resistance/1 -> Add/1
  Add/1 -> Inductancce/1
  Inductancce/1 -> Integrator/1
  Inertia/1 -> Integrator1/1
  Kt/1 -> Add1/1
  Add1/1 -> Inertia/1
  Integrator/1 -> Kt/1, Resistance/1
  Voltage/1 -> Add/2
  Dampling/1 -> Add1/2
  Integrator1/1 -> Dampling/1, Speed/1, Ke/1
  Ke/1 -> Add/3

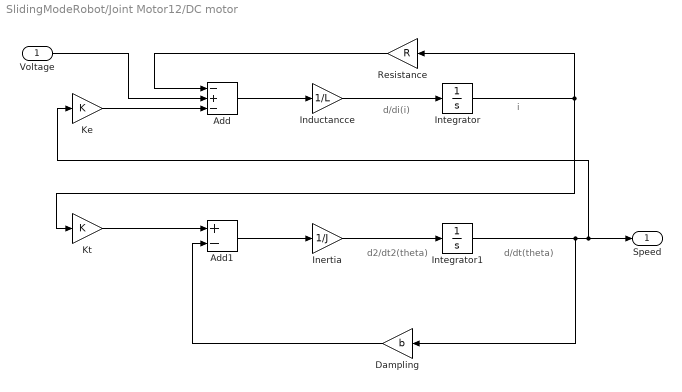
== system SlidingModeRobot/Joint Motor12/DC motor ==
  note: d/dt(theta)
  note: d2/dt2(theta)
  note: i
  note: d/di(i)
  Voltage : Inport
  Add : Sum  Inputs=-+-
  Add1 : Sum  Inputs=+-
  Dampling : Gain  Gain=b
  Inductancce : Gain  Gain=1/L
  Inertia : Gain  Gain=1/J
  Integrator : Integrator
  Integrator1 : Integrator
  Ke : Gain  Gain=K
  Kt : Gain  Gain=K
  Resistance : Gain  Gain=R
  Speed : Outport
  wires:
  Resistance/1 -> Add/1
  Add/1 -> Inductancce/1
  Inductancce/1 -> Integrator/1
  Inertia/1 -> Integrator1/1
  Kt/1 -> Add1/1
  Add1/1 -> Inertia/1
  Integrator/1 -> Kt/1, Resistance/1
  Voltage/1 -> Add/2
  Dampling/1 -> Add1/2
  Integrator1/1 -> Dampling/1, Speed/1, Ke/1
  Ke/1 -> Add/3

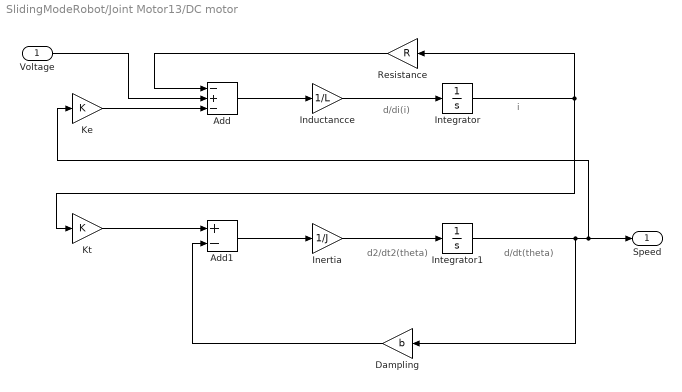
== system SlidingModeRobot/Joint Motor13/DC motor ==
  note: d/dt(theta)
  note: d2/dt2(theta)
  note: i
  note: d/di(i)
  Voltage : Inport
  Add : Sum  Inputs=-+-
  Add1 : Sum  Inputs=+-
  Dampling : Gain  Gain=b
  Inductancce : Gain  Gain=1/L
  Inertia : Gain  Gain=1/J
  Integrator : Integrator
  Integrator1 : Integrator
  Ke : Gain  Gain=K
  Kt : Gain  Gain=K
  Resistance : Gain  Gain=R
  Speed : Outport
  wires:
  Resistance/1 -> Add/1
  Add/1 -> Inductancce/1
  Inductancce/1 -> Integrator/1
  Inertia/1 -> Integrator1/1
  Kt/1 -> Add1/1
  Add1/1 -> Inertia/1
  Integrator/1 -> Kt/1, Resistance/1
  Voltage/1 -> Add/2
  Dampling/1 -> Add1/2
  Integrator1/1 -> Dampling/1, Speed/1, Ke/1
  Ke/1 -> Add/3

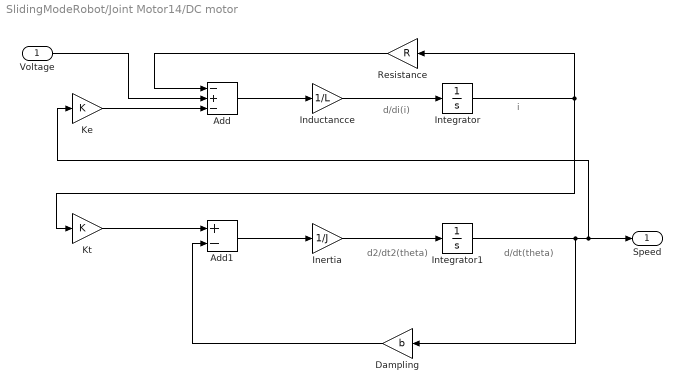
== system SlidingModeRobot/Joint Motor14/DC motor ==
  note: d/dt(theta)
  note: d2/dt2(theta)
  note: i
  note: d/di(i)
  Voltage : Inport
  Add : Sum  Inputs=-+-
  Add1 : Sum  Inputs=+-
  Dampling : Gain  Gain=b
  Inductancce : Gain  Gain=1/L
  Inertia : Gain  Gain=1/J
  Integrator : Integrator
  Integrator1 : Integrator
  Ke : Gain  Gain=K
  Kt : Gain  Gain=K
  Resistance : Gain  Gain=R
  Speed : Outport
  wires:
  Resistance/1 -> Add/1
  Add/1 -> Inductancce/1
  Inductancce/1 -> Integrator/1
  Inertia/1 -> Integrator1/1
  Kt/1 -> Add1/1
  Add1/1 -> Inertia/1
  Integrator/1 -> Kt/1, Resistance/1
  Voltage/1 -> Add/2
  Dampling/1 -> Add1/2
  Integrator1/1 -> Dampling/1, Speed/1, Ke/1
  Ke/1 -> Add/3

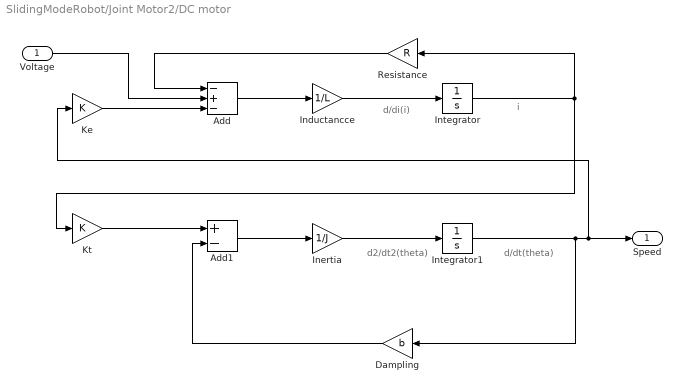
== system SlidingModeRobot/Joint Motor2/DC motor ==
  note: d/dt(theta)
  note: d2/dt2(theta)
  note: i
  note: d/di(i)
  Voltage : Inport
  Add : Sum  Inputs=-+-
  Add1 : Sum  Inputs=+-
  Dampling : Gain  Gain=b
  Inductancce : Gain  Gain=1/L
  Inertia : Gain  Gain=1/J
  Integrator : Integrator
  Integrator1 : Integrator
  Ke : Gain  Gain=K
  Kt : Gain  Gain=K
  Resistance : Gain  Gain=R
  Speed : Outport
  wires:
  Resistance/1 -> Add/1
  Add/1 -> Inductancce/1
  Inductancce/1 -> Integrator/1
  Inertia/1 -> Integrator1/1
  Kt/1 -> Add1/1
  Add1/1 -> Inertia/1
  Integrator/1 -> Kt/1, Resistance/1
  Voltage/1 -> Add/2
  Dampling/1 -> Add1/2
  Integrator1/1 -> Dampling/1, Speed/1, Ke/1
  Ke/1 -> Add/3

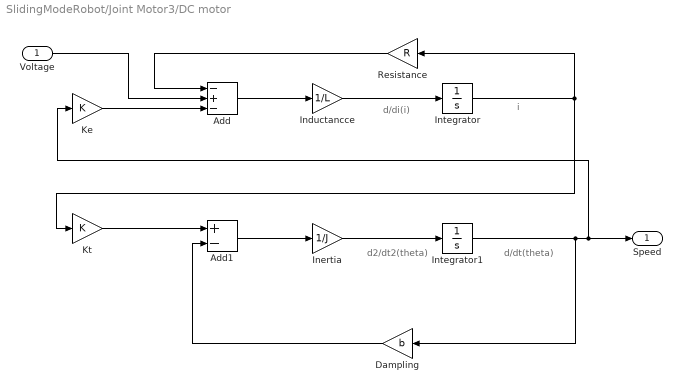
== system SlidingModeRobot/Joint Motor3/DC motor ==
  note: d/dt(theta)
  note: d2/dt2(theta)
  note: i
  note: d/di(i)
  Voltage : Inport
  Add : Sum  Inputs=-+-
  Add1 : Sum  Inputs=+-
  Dampling : Gain  Gain=b
  Inductancce : Gain  Gain=1/L
  Inertia : Gain  Gain=1/J
  Integrator : Integrator
  Integrator1 : Integrator
  Ke : Gain  Gain=K
  Kt : Gain  Gain=K
  Resistance : Gain  Gain=R
  Speed : Outport
  wires:
  Resistance/1 -> Add/1
  Add/1 -> Inductancce/1
  Inductancce/1 -> Integrator/1
  Inertia/1 -> Integrator1/1
  Kt/1 -> Add1/1
  Add1/1 -> Inertia/1
  Integrator/1 -> Kt/1, Resistance/1
  Voltage/1 -> Add/2
  Dampling/1 -> Add1/2
  Integrator1/1 -> Dampling/1, Speed/1, Ke/1
  Ke/1 -> Add/3

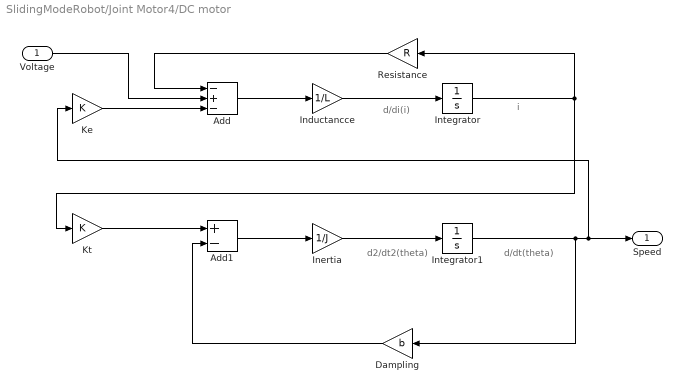
== system SlidingModeRobot/Joint Motor4/DC motor ==
  note: d/dt(theta)
  note: d2/dt2(theta)
  note: i
  note: d/di(i)
  Voltage : Inport
  Add : Sum  Inputs=-+-
  Add1 : Sum  Inputs=+-
  Dampling : Gain  Gain=b
  Inductancce : Gain  Gain=1/L
  Inertia : Gain  Gain=1/J
  Integrator : Integrator
  Integrator1 : Integrator
  Ke : Gain  Gain=K
  Kt : Gain  Gain=K
  Resistance : Gain  Gain=R
  Speed : Outport
  wires:
  Resistance/1 -> Add/1
  Add/1 -> Inductancce/1
  Inductancce/1 -> Integrator/1
  Inertia/1 -> Integrator1/1
  Kt/1 -> Add1/1
  Add1/1 -> Inertia/1
  Integrator/1 -> Kt/1, Resistance/1
  Voltage/1 -> Add/2
  Dampling/1 -> Add1/2
  Integrator1/1 -> Dampling/1, Speed/1, Ke/1
  Ke/1 -> Add/3

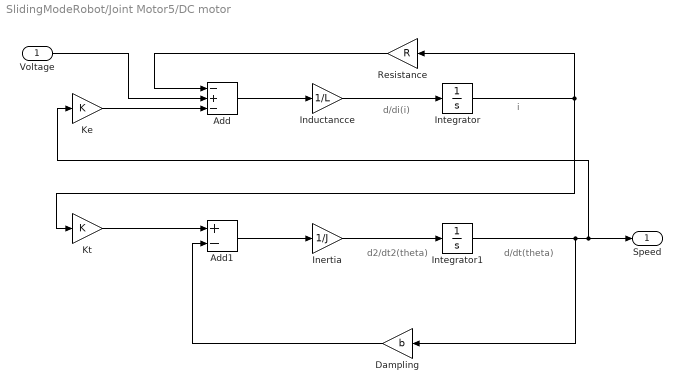
== system SlidingModeRobot/Joint Motor5/DC motor ==
  note: d/dt(theta)
  note: d2/dt2(theta)
  note: i
  note: d/di(i)
  Voltage : Inport
  Add : Sum  Inputs=-+-
  Add1 : Sum  Inputs=+-
  Dampling : Gain  Gain=b
  Inductancce : Gain  Gain=1/L
  Inertia : Gain  Gain=1/J
  Integrator : Integrator
  Integrator1 : Integrator
  Ke : Gain  Gain=K
  Kt : Gain  Gain=K
  Resistance : Gain  Gain=R
  Speed : Outport
  wires:
  Resistance/1 -> Add/1
  Add/1 -> Inductancce/1
  Inductancce/1 -> Integrator/1
  Inertia/1 -> Integrator1/1
  Kt/1 -> Add1/1
  Add1/1 -> Inertia/1
  Integrator/1 -> Kt/1, Resistance/1
  Voltage/1 -> Add/2
  Dampling/1 -> Add1/2
  Integrator1/1 -> Dampling/1, Speed/1, Ke/1
  Ke/1 -> Add/3

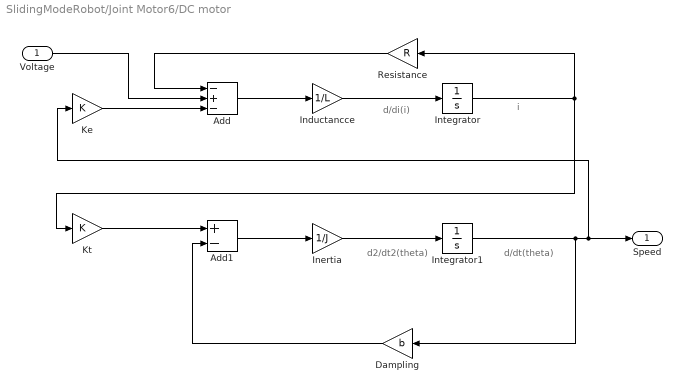
== system SlidingModeRobot/Joint Motor6/DC motor ==
  note: d/dt(theta)
  note: d2/dt2(theta)
  note: i
  note: d/di(i)
  Voltage : Inport
  Add : Sum  Inputs=-+-
  Add1 : Sum  Inputs=+-
  Dampling : Gain  Gain=b
  Inductancce : Gain  Gain=1/L
  Inertia : Gain  Gain=1/J
  Integrator : Integrator
  Integrator1 : Integrator
  Ke : Gain  Gain=K
  Kt : Gain  Gain=K
  Resistance : Gain  Gain=R
  Speed : Outport
  wires:
  Resistance/1 -> Add/1
  Add/1 -> Inductancce/1
  Inductancce/1 -> Integrator/1
  Inertia/1 -> Integrator1/1
  Kt/1 -> Add1/1
  Add1/1 -> Inertia/1
  Integrator/1 -> Kt/1, Resistance/1
  Voltage/1 -> Add/2
  Dampling/1 -> Add1/2
  Integrator1/1 -> Dampling/1, Speed/1, Ke/1
  Ke/1 -> Add/3

== system SlidingModeRobot/Joint Motor7/DC motor ==
  note: d/dt(theta)
  note: d2/dt2(theta)
  note: i
  note: d/di(i)
  Voltage : Inport
  Add : Sum  Inputs=-+-
  Add1 : Sum  Inputs=+-
  Dampling : Gain  Gain=b
  Inductancce : Gain  Gain=1/L
  Inertia : Gain  Gain=1/J
  Integrator : Integrator
  Integrator1 : Integrator
  Ke : Gain  Gain=K
  Kt : Gain  Gain=K
  Resistance : Gain  Gain=R
  Speed : Outport
  wires:
  Resistance/1 -> Add/1
  Add/1 -> Inductancce/1
  Inductancce/1 -> Integrator/1
  Inertia/1 -> Integrator1/1
  Kt/1 -> Add1/1
  Add1/1 -> Inertia/1
  Integrator/1 -> Kt/1, Resistance/1
  Voltage/1 -> Add/2
  Dampling/1 -> Add1/2
  Integrator1/1 -> Dampling/1, Speed/1, Ke/1
  Ke/1 -> Add/3

== system SlidingModeRobot/Joint Motor8/DC motor ==
  note: d/dt(theta)
  note: d2/dt2(theta)
  note: i
  note: d/di(i)
  Voltage : Inport
  Add : Sum  Inputs=-+-
  Add1 : Sum  Inputs=+-
  Dampling : Gain  Gain=b
  Inductancce : Gain  Gain=1/L
  Inertia : Gain  Gain=1/J
  Integrator : Integrator
  Integrator1 : Integrator
  Ke : Gain  Gain=K
  Kt : Gain  Gain=K
  Resistance : Gain  Gain=R
  Speed : Outport
  wires:
  Resistance/1 -> Add/1
  Add/1 -> Inductancce/1
  Inductancce/1 -> Integrator/1
  Inertia/1 -> Integrator1/1
  Kt/1 -> Add1/1
  Add1/1 -> Inertia/1
  Integrator/1 -> Kt/1, Resistance/1
  Voltage/1 -> Add/2
  Dampling/1 -> Add1/2
  Integrator1/1 -> Dampling/1, Speed/1, Ke/1
  Ke/1 -> Add/3

== system SlidingModeRobot/Joint Motor9/DC motor ==
  note: d/dt(theta)
  note: d2/dt2(theta)
  note: i
  note: d/di(i)
  Voltage : Inport
  Add : Sum  Inputs=-+-
  Add1 : Sum  Inputs=+-
  Dampling : Gain  Gain=b
  Inductancce : Gain  Gain=1/L
  Inertia : Gain  Gain=1/J
  Integrator : Integrator
  Integrator1 : Integrator
  Ke : Gain  Gain=K
  Kt : Gain  Gain=K
  Resistance : Gain  Gain=R
  Speed : Outport
  wires:
  Resistance/1 -> Add/1
  Add/1 -> Inductancce/1
  Inductancce/1 -> Integrator/1
  Inertia/1 -> Integrator1/1
  Kt/1 -> Add1/1
  Add1/1 -> Inertia/1
  Integrator/1 -> Kt/1, Resistance/1
  Voltage/1 -> Add/2
  Dampling/1 -> Add1/2
  Integrator1/1 -> Dampling/1, Speed/1, Ke/1
  Ke/1 -> Add/3
